simulink model "adaptive_control"  (R2023b)
settings: Solver=VariableStepAuto  StartTime=0.0  StopTime=60  RelTol=1e-5
values from neighbouring files (symbols this model uses):
  A = Ixx-Kpdot    (= 4100300)    [ShipFinStabilizers.m]
  alpha = 200    [ShipFinStabilizers.m]
  Am = [0,1;-1.412, -1.0259]    [ShipFinStabilizers.m]
  B = Kp + Kup - 2*Kalpha*rf/U    (= -505089.3115)    [ShipFinStabilizers.m]
  beta = 100    [ShipFinStabilizers.m]
  Bm = [0;1]    [ShipFinStabilizers.m]
  C = Knl    (= -416000)    [ShipFinStabilizers.m]
  D = KphiUU*U^2    (= -265500)    [ShipFinStabilizers.m]
  F = -2*Kalpha    (= -18034.875)    [ShipFinStabilizers.m]
  Fw = 0.2    [ShipFinStabilizers.m]    (also in plotRoutine.m = Fw_vect(i))
  omega_w = 1.3    [ShipFinStabilizers.m]    (also in plotRoutine.m = omega_w_vect(j))
  sat = 45    [ShipFinStabilizers.m]
  x0 = [deg2rad(20);0]    [ShipFinStabilizers.m]
PauseFcn:
  | e1.m
settings Model: Creator=valen  LastModifiedBy=valen

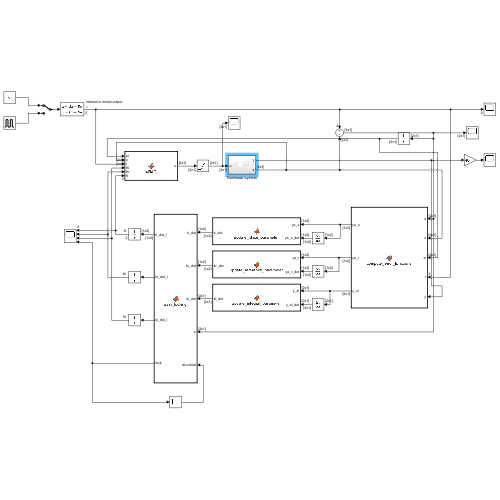
[thumbnail: Simulink's stored preview of the top-level diagram]
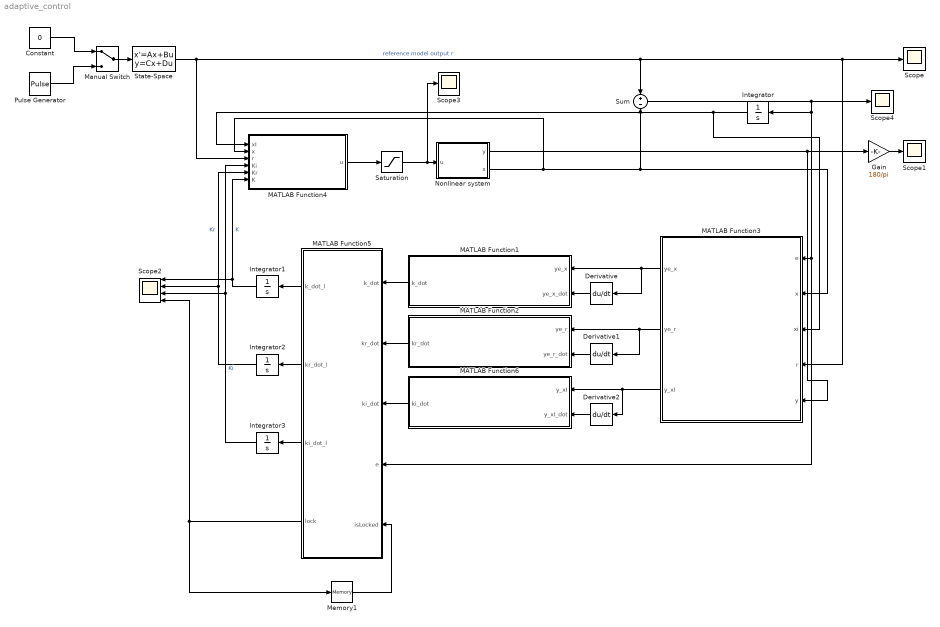
== system adaptive_control ==
  Constant : Constant  Value=0
  Derivative : Derivative
  Derivative1 : Derivative
  Derivative2 : Derivative
  Gain : Gain  Gain=180/pi
  Integrator : Integrator
  Integrator1 : Integrator  InitialCondition=[0,0]
  Integrator2 : Integrator
  Integrator3 : Integrator
  MATLAB Function1 : MATLAB Function  TreatAsAtomicUnit=on
  MATLAB Function2 : MATLAB Function  TreatAsAtomicUnit=on
  MATLAB Function3 : MATLAB Function  TreatAsAtomicUnit=on
  MATLAB Function4 : MATLAB Function  TreatAsAtomicUnit=on
  MATLAB Function5 : MATLAB Function  TreatAsAtomicUnit=on
  MATLAB Function6 : MATLAB Function  TreatAsAtomicUnit=on
  Manual Switch : ManualSwitch
  Memory1 : Memory
  Nonlinear system : Subsystem
  Pulse Generator : DiscretePulseGenerator  PulseType=Time based  Period=20  PulseWidth=80
  Saturation : Saturate  UpperLimit=sat  LowerLimit=-sat
  Scope{,1,3..4} (4 alike) : Scope
  Scope2 : Scope  NumInputPorts=4
  State-Space : StateSpace  A=Am  B=Bm  C=eye(2)  D=[0;0]  InitialCondition=x0
  Sum : Sum  Inputs=+-
  wires:
  State-Space/1 -> MATLAB Function4/3(r), MATLAB Function3/4(r), Scope/1, Sum/1  "reference model output r"
  MATLAB Function3/1(ye_x) -> Derivative/1, MATLAB Function1/1(ye_x)
  MATLAB Function3/2(ye_r) -> Derivative1/1, MATLAB Function2/1(ye_r)
  Derivative/1 -> MATLAB Function1/2(ye_x_dot)
  Derivative1/1 -> MATLAB Function2/2(ye_r_dot)
  Sum/1 -> MATLAB Function5/4(e), MATLAB Function3/1(e), Integrator/1, Scope4/1
  Integrator2/1 -> MATLAB Function4/5(Kr), Scope2/2  "Kr"
  Integrator1/1 -> MATLAB Function4/6(K), Scope2/1  "K"
  MATLAB Function4/1(u) -> Saturation/1
  Manual Switch/1 -> State-Space/1
  Constant/1 -> Manual Switch/1
  Pulse Generator/1 -> Manual Switch/2
  MATLAB Function2/1(kr_dot) -> MATLAB Function5/2(kr_dot)
  MATLAB Function1/1(k_dot) -> MATLAB Function5/1(k_dot)
  MATLAB Function5/1(k_dot_l) -> Integrator1/1
  MATLAB Function5/2(kr_dot_l) -> Integrator2/1
  MATLAB Function5/4(lock) -> Memory1/1, Scope2/4
  Nonlinear system/2(x) -> MATLAB Function4/2(x), Sum/2, MATLAB Function3/2(x)
  Nonlinear system/1(y) -> MATLAB Function3/5(y), Gain/1
  Gain/1 -> Scope1/1
  Saturation/1 -> Scope3/1, Nonlinear system/1(u)
  Integrator/1 -> MATLAB Function3/3(xi), MATLAB Function4/1(xI)
  MATLAB Function3/3(y_xI) -> Derivative2/1, MATLAB Function6/1(y_xI)
  Derivative2/1 -> MATLAB Function6/2(y_xI_dot)
  MATLAB Function6/1(ki_dot) -> MATLAB Function5/3(ki_dot)
  MATLAB Function5/3(ki_dot_l) -> Integrator3/1
  Integrator3/1 -> Scope2/3, MATLAB Function4/4(Ki)  "Ki"
  Memory1/1 -> MATLAB Function5/5(isLocked)

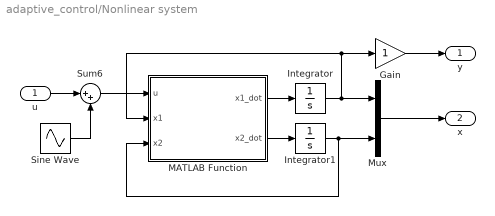
== system adaptive_control/Nonlinear system ==
  u : Inport
  Gain : Gain
  Integrator : Integrator  InitialCondition=x0(1)
  Integrator1 : Integrator  InitialCondition=x0(2)
  MATLAB Function : MATLAB Function  TreatAsAtomicUnit=on
  Mux : Mux  Inputs=2
  Sine Wave : Sin  Amplitude=Fw/F*A  Frequency=omega_w  SampleTime=0
  Sum6 : Sum  Inputs=|++
  y : Outport
  x : Outport  Port=2  PortDimensions=[2;1]
  wires:
  Integrator1/1 -> Mux/2, MATLAB Function/3(x2)
  Integrator/1 -> Mux/1, Gain/1, MATLAB Function/2(x1)
  MATLAB Function/2(x2_dot) -> Integrator1/1
  MATLAB Function/1(x1_dot) -> Integrator/1
  Mux/1 -> x/1
  Sine Wave/1 -> Sum6/2
  u/1 -> Sum6/1
  Sum6/1 -> MATLAB Function/1(u)
  Gain/1 -> y/1

== matlab function adaptive_control/MATLAB Function1 ==
  data: ye_x input; k_dot output; ye_x_dot input; alpha parameter; beta parameter
function k_dot = update_state_parameter(ye_x, ye_x_dot, alpha, beta)


k_dot = alpha*ye_x + beta *ye_x_dot;

== matlab function adaptive_control/Nonlinear system/MATLAB Function ==
  data: u input; x1_dot output; x1 input; x2 input; x2_dot output; A parameter; B parameter; C parameter; D parameter; E parameter; F parameter
function [x1_dot,x2_dot] = ship(u,x1,x2, A, B, C, D, E, F)

    x1_dot = x2;
    x2_dot = 1/A*( B*x2 + C*x2*abs(x2) + D*x1 + E*sin(x1) + F*u);

== matlab function adaptive_control/MATLAB Function2 ==
  data: ye_r input; kr_dot output; ye_r_dot input; alpha parameter; beta parameter
function kr_dot = update_reference_parameter(ye_r, ye_r_dot, alpha, beta)


kr_dot = alpha*ye_r + beta *ye_r_dot;

== matlab function adaptive_control/MATLAB Function3 ==
  data: e input; x input; xi input; r input; y input; ye_x output; ye_r output; Ce parameter; y_xI output
function [ye_x, ye_r,y_xI] = compute_error_functions(e, x, xi,r, y, Ce)

ye_x = Ce*e*x';
ye_r = Ce*e*r';
y_xI = y*xi;

== matlab function adaptive_control/MATLAB Function4 ==
  data: xI input; x input size=[2;1]; r input; Ki input; Kr input; K input; u output
function u = MRAC(xI, x, r,Ki, Kr, K)

u = Kr*r + K(1)*x(1) + K(2)*x(2) +Ki*xI;

== matlab function adaptive_control/MATLAB Function5 ==
  data: k_dot input; k_dot_l output; kr_dot input; ki_dot input; e input; kr_dot_l output; ki_dot_l output; lock output; isLocked input
function [k_dot_l, kr_dot_l,ki_dot_l, lock] = gain_locking(k_dot,kr_dot, ki_dot,e, isLocked)


if norm(e) < 1e-3 || isLocked
    k_dot_l = zeros(1,2);
    kr_dot_l = 0;
    ki_dot_l = 0;
    lock = 1;
else
    k_dot_l = k_dot;
    kr_dot_l = kr_dot;
    ki_dot_l = ki_dot;
    lock = 0;
end

== matlab function adaptive_control/MATLAB Function6 ==
  data: y_xI input; ki_dot output; y_xI_dot input; alpha parameter; beta parameter
function ki_dot = update_integral_parameter(y_xI, y_xI_dot,alpha, beta)


ki_dot = alpha*y_xI + beta*y_xI_dot;
